simulink model "simulink_run"  (R2014b)
settings: Solver=ode3  StartTime=0.0  StopTime=72.0  FixedStep=0.001  RelTol=1e-3
settings Model: Creator=root  LastModifiedBy=root

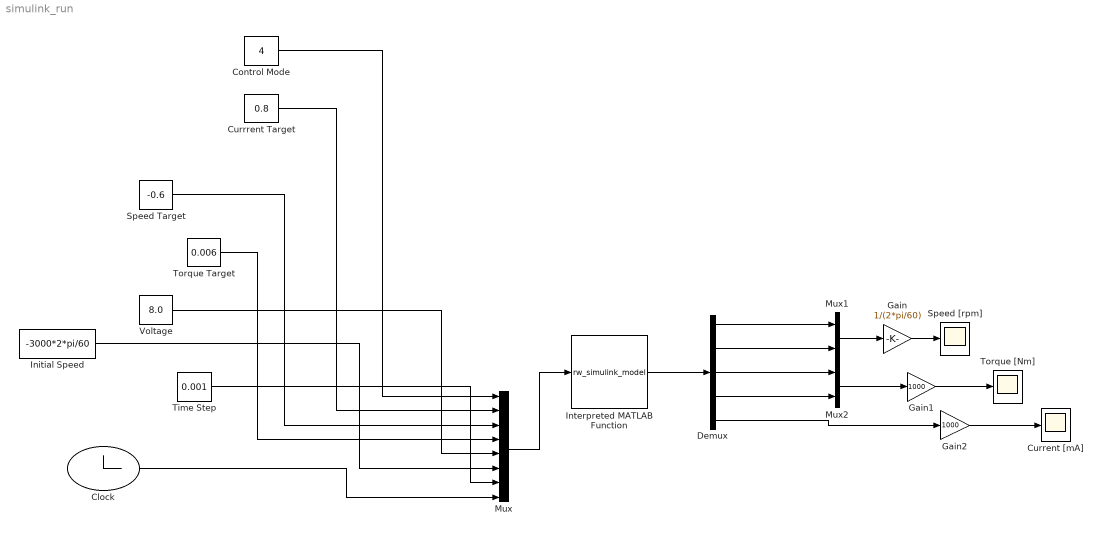
== system simulink_run ==
  Clock : Clock
      settings: Decimation=1000
  Control Mode : Constant  Value=4
  Current [mA] : Scope
      settings: TimeRange=50  YMin=-1000  YMax=1000  SaveName=ScopeData2
  Currrent Target : Constant  Value=0.8
  Demux : Demux  Outputs=5
  Gain : Gain  Gain=1/(2*pi/60)
  Gain1 : Gain  Gain=1000
  Gain2 : Gain  Gain=1000
  Initial Speed : Constant  Value=-3000*2*pi/60
  Interpreted MATLAB Function : MATLABFcn  MATLABFcn=rw_simulink_model  OutputDimensions=5
  Mux : Mux  Inputs=8
  Mux1 : Mux  Inputs=2
  Mux2 : Mux  Inputs=2
  Speed Target : Constant  Value=-0.6
  Speed [rpm] : Scope
      settings: TimeRange=50  YMin=-3000  YMax=-2000
  Time Step : Constant  Value=0.001
  Torque Target : Constant  Value=0.006
  Torque [Nm] : Scope
      settings: TimeRange=50  YMin=-30  YMax=30
  Voltage : Constant  Value=8.0
  wires:
  Clock/1 -> Mux/8
  Control Mode/1 -> Mux/1
  Mux/1 -> Interpreted MATLAB Function/1
  Currrent Target/1 -> Mux/2
  Speed Target/1 -> Mux/3
  Torque Target/1 -> Mux/4
  Voltage/1 -> Mux/5
  Initial Speed/1 -> Mux/6
  Time Step/1 -> Mux/7
  Interpreted MATLAB Function/1 -> Demux/1
  Mux1/1 -> Gain/1
  Gain/1 -> Speed [rpm]/1
  Demux/1 -> Mux1/1
  Demux/2 -> Mux1/2
  Demux/3 -> Mux2/1
  Demux/4 -> Mux2/2
  Mux2/1 -> Gain1/1
  Gain1/1 -> Torque [Nm]/1
  Demux/5 -> Gain2/1
  Gain2/1 -> Current [mA]/1
